simulink model "pmsm"  (R2018a)
settings: Solver=FixedStepDiscrete  StartTime=0.0  StopTime=0.4  RelTol=1e-3
libraries: powerlib x13
settings Model: Creator=R-YDL  LastModifiedBy=R-YDL

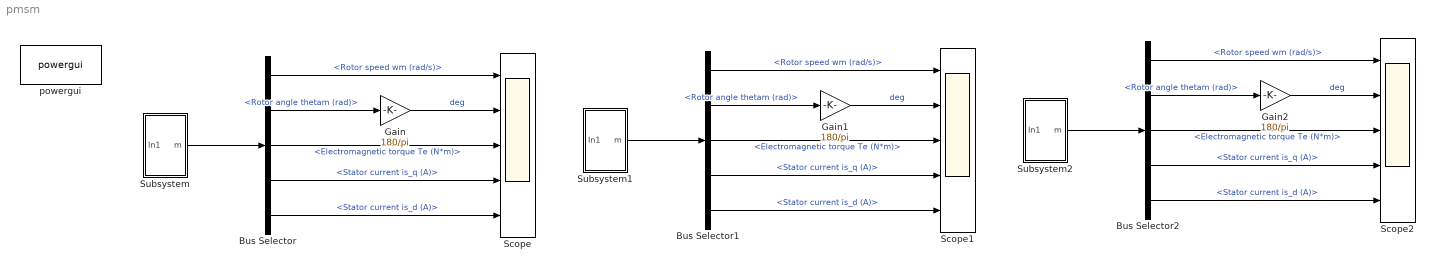
== system pmsm ==
  Bus Selector : BusSelector  OutputSignals=Rotor speed wm (rad/s),Rotor angle thetam (rad),Electromagnetic torque Te (N*m),Stator current is_q (A),Stator current is_d (A)
  Bus Selector1 : BusSelector  OutputSignals=Rotor speed wm (rad/s),Rotor angle thetam (rad),Electromagnetic torque Te (N*m),Stator current is_q (A),Stator current is_d (A)
  Bus Selector2 : BusSelector  OutputSignals=Rotor speed wm (rad/s),Rotor angle thetam (rad),Electromagnetic torque Te (N*m),Stator current is_q (A),Stator current is_d (A)
  Gain : Gain  Gain=180/pi
  Gain1 : Gain  Gain=180/pi
  Gain2 : Gain  Gain=180/pi
  Scope : Scope  NumInputPorts=5
  Scope1 : Scope  NumInputPorts=5
  Scope2 : Scope  NumInputPorts=5
  Subsystem : Subsystem  mask{Va=20, Vb=0, Vc=0, t0=0}
  Subsystem1 : Subsystem  mask{Va=20, Vb=20, Vc=0, t0=0}
  Subsystem2 : Subsystem  mask{Va=0, Vb=20, Vc=0, t0=60}
  powergui : powerlib/powergui  Priority=1  SimulationMode=Discrete  SampleTime=2e-6  frequency=60  Iterations=50  frequencyindice=0  Pbase=100e6  ErrMax=1e-4  UnitsV=kV  UnitsW=MW  buscounter=0  FunctionMessages=off  echomessages=off  EnableUseOfTLC=off  CurrentSourceSwitches=off  DisableSnubberDevices=off  DisableRonSwitches=off  DisableVfSwitches=off  DisplayEquations=off  SolverType=Tustin/Backward Euler (TBE)  Interpol=off  ExternalGateDelay=off  methode=off  Ts=100  x0status=blocks  SPID=on  SwTol=0  HookPort=off  RestoreLinks=warning  ResistiveCurrentMeasurement=off  Frange=[0:2:500]  Ylog=off  Xlog=on  ShowGrid=off  save=off  variable=ZData  structure=0  ZoomFFT=off  StartTime=0.0  cycles=1  DisplayStyle=1  fundamental=60  FreqAxis=off  MaxFrequency=1000  frequencyindicesteady=1  RmsSteady=1  display=off
  wires:
  Bus Selector/1 -> Scope/1  "<Rotor speed wm (rad/s)>"
  Bus Selector/2 -> Gain/1  "<Rotor angle thetam (rad)>"
  Bus Selector/3 -> Scope/3  "<Electromagnetic torque Te (N*m)>"
  Bus Selector/4 -> Scope/4  "<Stator current is_q (A)>"
  Bus Selector/5 -> Scope/5  "<Stator current is_d (A)>"
  Gain/1 -> Scope/2  "deg"
  Subsystem/1(m) -> Bus Selector/1
  Subsystem1/1(m) -> Bus Selector1/1
  Bus Selector1/2 -> Gain1/1  "<Rotor angle thetam (rad)>"
  Gain1/1 -> Scope1/2  "deg"
  Bus Selector1/4 -> Scope1/4  "<Stator current is_q (A)>"
  Bus Selector1/5 -> Scope1/5  "<Stator current is_d (A)>"
  Bus Selector1/1 -> Scope1/1  "<Rotor speed wm (rad/s)>"
  Bus Selector1/3 -> Scope1/3  "<Electromagnetic torque Te (N*m)>"
  Bus Selector2/1 -> Scope2/1  "<Rotor speed wm (rad/s)>"
  Bus Selector2/4 -> Scope2/4  "<Stator current is_q (A)>"
  Bus Selector2/5 -> Scope2/5  "<Stator current is_d (A)>"
  Subsystem2/1(m) -> Bus Selector2/1
  Bus Selector2/3 -> Scope2/3  "<Electromagnetic torque Te (N*m)>"
  Gain2/1 -> Scope2/2  "deg"
  Bus Selector2/2 -> Gain2/1  "<Rotor angle thetam (rad)>"

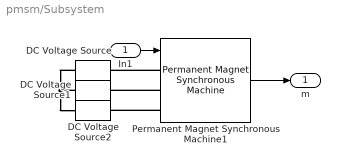
== system pmsm/Subsystem ==
  In1 : Inport
  DC Voltage Source : powerlib/Electrical Sources/DC Voltage Source  Amplitude=Va  Measurements=None
  DC Voltage Source1 : powerlib/Electrical Sources/DC Voltage Source  Amplitude=Vb  Measurements=None
  DC Voltage Source2 : powerlib/Electrical Sources/DC Voltage Source  Amplitude=Vc  Measurements=None
  Permanent Magnet Synchronous Machine1 : powerlib/Machines/Permanent Magnet Synchronous Machine  NbPhases=3  FluxDistribution=Sinusoidal  RotorType=Round  MechanicalLoad=Torque Tm  PresetModel=No  ShowDetailedParameters=on  MeasurementBus=off  Resistance=0.0485  Inductance=8.5e-3  dqInductances=[8.5e-3,8.5e-3]  La=0.000395  MachineConstant=Flux linkage established by magnets (V.s)  Flux=0.1194  VoltageCst=21.6568  TorqueCst=0.1791  Flat=120  Mechanical=[0.0027 0.0424924 1 0]  PolePairs=4  InitialConditions=[0,t0, 0,0]  InitialConditions5ph=[0 0 0 0 0 0]  TsPowergui=0  TsBlock=-1  RefAngle=Aligned with phase A axis (original Park)
      settings: SourceProductName=Simscape Power Systems
  m : Outport
  wires:
  In1/1 -> Permanent Magnet Synchronous Machine1/1
  Permanent Magnet Synchronous Machine1/1 -> m/1
  connections:
  Permanent Magnet Synchronous Machine1/LConn1 -- DC Voltage Source/RConn1
  Permanent Magnet Synchronous Machine1/LConn2 -- DC Voltage Source1/RConn1
  DC Voltage Source/LConn1 -- DC Voltage Source1/LConn1 -- DC Voltage Source2/LConn1
  Permanent Magnet Synchronous Machine1/LConn3 -- DC Voltage Source2/RConn1

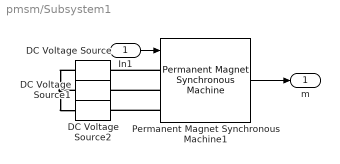
== system pmsm/Subsystem1 ==
  In1 : Inport
  DC Voltage Source : powerlib/Electrical Sources/DC Voltage Source  Amplitude=Va  Measurements=None
  DC Voltage Source1 : powerlib/Electrical Sources/DC Voltage Source  Amplitude=Vb  Measurements=None
  DC Voltage Source2 : powerlib/Electrical Sources/DC Voltage Source  Amplitude=Vc  Measurements=None
  Permanent Magnet Synchronous Machine1 : powerlib/Machines/Permanent Magnet Synchronous Machine  NbPhases=3  FluxDistribution=Sinusoidal  RotorType=Round  MechanicalLoad=Torque Tm  PresetModel=No  ShowDetailedParameters=on  MeasurementBus=off  Resistance=0.0485  Inductance=8.5e-3  dqInductances=[8.5e-3,8.5e-3]  La=0.000395  MachineConstant=Flux linkage established by magnets (V.s)  Flux=0.1194  VoltageCst=21.6568  TorqueCst=0.1791  Flat=120  Mechanical=[0.0027 0.0424924 1 0]  PolePairs=4  InitialConditions=[0,t0, 0,0]  InitialConditions5ph=[0 0 0 0 0 0]  TsPowergui=0  TsBlock=-1  RefAngle=Aligned with phase A axis (original Park)
      settings: SourceProductName=Simscape Power Systems
  m : Outport
  wires:
  In1/1 -> Permanent Magnet Synchronous Machine1/1
  Permanent Magnet Synchronous Machine1/1 -> m/1
  connections:
  Permanent Magnet Synchronous Machine1/LConn1 -- DC Voltage Source/RConn1
  Permanent Magnet Synchronous Machine1/LConn2 -- DC Voltage Source1/RConn1
  DC Voltage Source/LConn1 -- DC Voltage Source2/LConn1 -- DC Voltage Source1/LConn1
  Permanent Magnet Synchronous Machine1/LConn3 -- DC Voltage Source2/RConn1

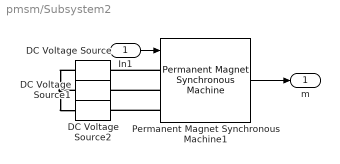
== system pmsm/Subsystem2 ==
  In1 : Inport
  DC Voltage Source : powerlib/Electrical Sources/DC Voltage Source  Amplitude=Va  Measurements=None
  DC Voltage Source1 : powerlib/Electrical Sources/DC Voltage Source  Amplitude=Vb  Measurements=None
  DC Voltage Source2 : powerlib/Electrical Sources/DC Voltage Source  Amplitude=Vc  Measurements=None
  Permanent Magnet Synchronous Machine1 : powerlib/Machines/Permanent Magnet Synchronous Machine  NbPhases=3  FluxDistribution=Sinusoidal  RotorType=Round  MechanicalLoad=Torque Tm  PresetModel=No  ShowDetailedParameters=on  MeasurementBus=off  Resistance=0.0485  Inductance=8.5e-3  dqInductances=[8.5e-3,8.5e-3]  La=0.000395  MachineConstant=Flux linkage established by magnets (V.s)  Flux=0.1194  VoltageCst=21.6568  TorqueCst=0.1791  Flat=120  Mechanical=[0.0027 0.0424924 1 0]  PolePairs=4  InitialConditions=[0,t0, 0,0]  InitialConditions5ph=[0 0 0 0 0 0]  TsPowergui=0  TsBlock=-1  RefAngle=Aligned with phase A axis (original Park)
      settings: SourceProductName=Simscape Power Systems
  m : Outport
  wires:
  In1/1 -> Permanent Magnet Synchronous Machine1/1
  Permanent Magnet Synchronous Machine1/1 -> m/1
  connections:
  Permanent Magnet Synchronous Machine1/LConn1 -- DC Voltage Source/RConn1
  Permanent Magnet Synchronous Machine1/LConn2 -- DC Voltage Source1/RConn1
  DC Voltage Source/LConn1 -- DC Voltage Source2/LConn1 -- DC Voltage Source1/LConn1
  Permanent Magnet Synchronous Machine1/LConn3 -- DC Voltage Source2/RConn1
